simulink model "Modulador_Analogico_CuatroUsuarios"  (R2018b)
settings: Solver=FixedStepAuto  StartTime=0.0  StopTime=M*CantBit  FixedStep=Tsampling  RelTol=1e-3
values from neighbouring files (symbols this model uses):
  CantMPerSimbOFDM = round(TsOFDM/Tsampling)    [Script_configParametros.m]
  EsOFDM = 2    [Script_configParametros.m]
  F1 = FsepOFDM*2    [Script_configParametros.m]
  F2 = FsepOFDM*3    [Script_configParametros.m]
  F3 = FsepOFDM*4    [Script_configParametros.m]
  F4 = FsepOFDM*5    [Script_configParametros.m]
  Tb1 = 1/Rb1    (= 0.001)    [Script_configParametros.m]
  Tb2 = 1/Rb2    (= 0.001)    [Script_configParametros.m]
  Tb3 = 1/Rb3    (= 0.0005)    [Script_configParametros.m]
  Tb4 = 1/Rb4    (= 0.000333333333333)    [Script_configParametros.m]
  Ts1 = Tb1    (= 0.001)    [Script_configParametros.m]
  Ts2 = Tb2    (= 0.001)    [Script_configParametros.m]
  Ts3 = 2*Tb3    (= 0.001)    [Script_configParametros.m]
  Ts4 = 3*Tb4    (= 0.001)    [Script_configParametros.m]
  Tsampling = M/N    [Script_configParametros.m]
libraries: commdigbbndpm3 x4, commrandsrc3 x4
settings Model: Creator=lukit  LastModifiedBy=lukit

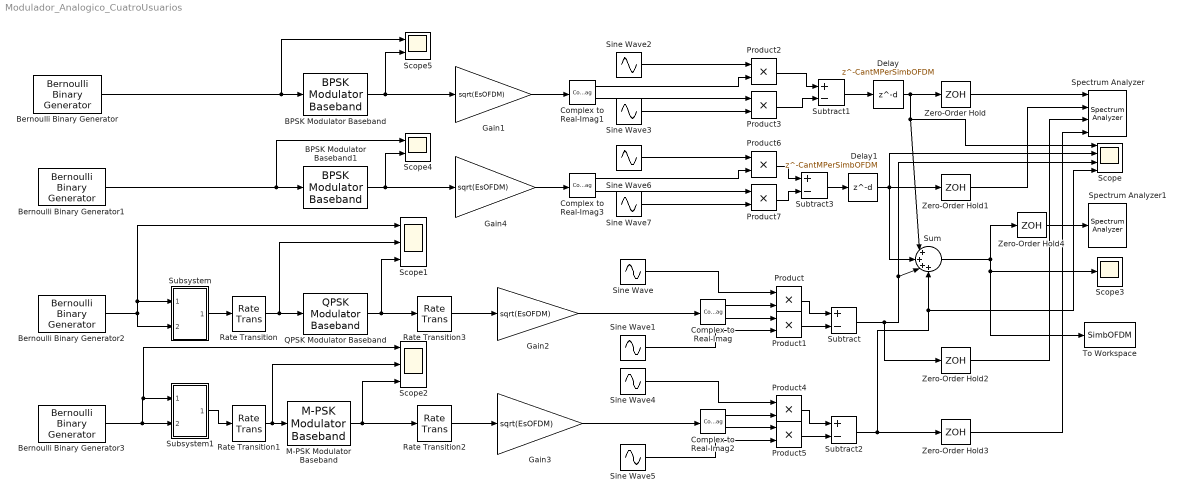
== system Modulador_Analogico_CuatroUsuarios ==
  BPSK Modulator Baseband : commdigbbndpm3/BPSK Modulator Baseband  Ph=0  outDtype=double  outWordLen=16  outUDDataType=sfix(16)  outFracLenMode=Best precision  outFracLen=15  outDataTypeStr=double  outLastDataTypeStr=double
  BPSK Modulator Baseband1 : commdigbbndpm3/BPSK Modulator Baseband  Ph=0  outDtype=double  outWordLen=16  outUDDataType=sfix(16)  outFracLenMode=Best precision  outFracLen=15  outDataTypeStr=double  outLastDataTypeStr=double
  Bernoulli Binary Generator : commrandsrc3/Bernoulli Binary Generator  ProbabilityOfZero=0.5  SeedSource=Auto  Seed=0  SampleTime=Tb1  SamplesPerFrame=1  OutputDataType=double  SimulateUsing=Interpreted execution
  Bernoulli Binary Generator1 : commrandsrc3/Bernoulli Binary Generator  ProbabilityOfZero=0.5  SeedSource=Auto  Seed=0  SampleTime=Tb2  SamplesPerFrame=1  OutputDataType=double  SimulateUsing=Interpreted execution
  Bernoulli Binary Generator2 : commrandsrc3/Bernoulli Binary Generator  ProbabilityOfZero=0.5  SeedSource=Auto  Seed=0  SampleTime=Tb3  SamplesPerFrame=1  OutputDataType=double  SimulateUsing=Interpreted execution
  Bernoulli Binary Generator3 : commrandsrc3/Bernoulli Binary Generator  ProbabilityOfZero=0.5  SeedSource=Auto  Seed=0  SampleTime=Tb4  SamplesPerFrame=1  OutputDataType=double  SimulateUsing=Interpreted execution
  Complex to Real-Imag{,1..3} (4 alike) : ComplexToRealImag
  Delay : Delay  DelayLength=CantMPerSimbOFDM  InitialCondition=0  SampleTime=Tsampling
  Delay1 : Delay  DelayLength=CantMPerSimbOFDM  InitialCondition=0  SampleTime=Tsampling
  Gain{1..4} (4 alike) : Gain  Gain=sqrt(EsOFDM)
  M-PSK Modulator Baseband : commdigbbndpm3/M-PSK Modulator Baseband  M=8  InType=Integer  Enc=Gray  Mapping=[0:7]  Ph=0  outDtype=double  outWordLen=16  outUDDataType=sfix(16)  outFracLenMode=Best precision  outFracLen=15  outDataTypeStr=double  outLastDataTypeStr=double
      settings: SourceProductName=Communications System Toolbox
  Product{,1..7} (8 alike) : Product
  QPSK Modulator Baseband : commdigbbndpm3/QPSK Modulator Baseband  InType=Integer  Enc=Gray  Ph=0  outDtype=double  outWordLen=16  outUDDataType=sfix(16)  outFracLenMode=Best precision  outFracLen=15  outDataTypeStr=double  outLastDataTypeStr=double
  Rate Transition : RateTransition  OutPortSampleTime=Ts3
  Rate Transition1 : RateTransition  OutPortSampleTime=Ts4
  Rate Transition2 : RateTransition  OutPortSampleTime=Tsampling
  Rate Transition3 : RateTransition  OutPortSampleTime=Tsampling
  Scope : Scope  NumInputPorts=4
  Scope1 : Scope  NumInputPorts=3
  Scope2 : Scope  NumInputPorts=3
  Scope3 : Scope
  Scope4 : Scope  NumInputPorts=2
  Scope5 : Scope  NumInputPorts=2
  Sine Wave : Sin  Amplitude=sqrt(2/Ts3)  Frequency=2*pi*F3  Phase=pi/2  SampleTime=Tsampling
  Sine Wave1 : Sin  Amplitude=sqrt(2/Ts3)  Frequency=2*pi*F3  SampleTime=Tsampling
  Sine Wave2 : Sin  Amplitude=sqrt(2/Ts1)  Frequency=2*pi*F1  Phase=pi/2  SampleTime=Tsampling
  Sine Wave3 : Sin  Amplitude=sqrt(2/Ts1)  Frequency=2*pi*F1  SampleTime=Tsampling
  Sine Wave4 : Sin  Amplitude=sqrt(2/Ts4)  Frequency=2*pi*F4  Phase=pi/2  SampleTime=Tsampling
  Sine Wave5 : Sin  Amplitude=sqrt(2/Ts4)  Frequency=2*pi*F4  SampleTime=Tsampling
  Sine Wave6 : Sin  Amplitude=sqrt(2/Ts2)  Frequency=2*pi*F2  Phase=pi/2  SampleTime=Tsampling
  Sine Wave7 : Sin  Amplitude=sqrt(2/Ts2)  Frequency=2*pi*F2  SampleTime=Tsampling
  Spectrum Analyzer : SpectrumAnalyzer  NumInputPorts=4
  Spectrum Analyzer1 : SpectrumAnalyzer
  Subsystem : Subsystem
  Subsystem1 : Subsystem
  Subtract{,1..3} (4 alike) : Sum  Inputs=+-
  Sum : Sum  Inputs=|++++
  To Workspace : ToWorkspace  VariableName=SimbOFDM  SampleTime=Tsampling
      settings: Save2DSignal=2-D array (concatenate along first dimension)
  Zero-Order Hold{,1..4} (5 alike) : ZeroOrderHold  SampleTime=-1
  wires:
  Product/1 -> Subtract/1
  Product1/1 -> Subtract/2
  Sine Wave/1 -> Product/1
  Sine Wave1/1 -> Product1/2
  Complex to Real-Imag/2 -> Product1/1
  Complex to Real-Imag/1 -> Product/2
  Gain2/1 -> Complex to Real-Imag/1
  Bernoulli Binary Generator/1 -> Scope5/1, BPSK Modulator Baseband/1
  Sine Wave2/1 -> Product2/1
  Complex to Real-Imag1/1 -> Product2/2
  Sine Wave3/1 -> Product3/2
  Complex to Real-Imag1/2 -> Product3/1
  Gain1/1 -> Complex to Real-Imag1/1
  Product2/1 -> Subtract1/1
  Product3/1 -> Subtract1/2
  BPSK Modulator Baseband/1 -> Scope5/2, Gain1/1
  Subtract/1 -> Zero-Order Hold2/1, Scope/3, Sum/3
  QPSK Modulator Baseband/1 -> Rate Transition3/1, Scope1/3
  M-PSK Modulator Baseband/1 -> Scope2/3, Rate Transition2/1
  Product4/1 -> Subtract2/1
  Sine Wave4/1 -> Product4/1
  Product5/1 -> Subtract2/2
  Sine Wave5/1 -> Product5/2
  Subtract2/1 -> Zero-Order Hold3/1, Scope/4, Sum/4
  Complex to Real-Imag2/2 -> Product5/1
  Complex to Real-Imag2/1 -> Product4/2
  Gain3/1 -> Complex to Real-Imag2/1
  Bernoulli Binary Generator1/1 -> Scope4/1, BPSK Modulator Baseband1/1
  BPSK Modulator Baseband1/1 -> Scope4/2, Gain4/1
  Sine Wave6/1 -> Product6/1
  Complex to Real-Imag3/1 -> Product6/2
  Sine Wave7/1 -> Product7/2
  Product6/1 -> Subtract3/1
  Product7/1 -> Subtract3/2
  Complex to Real-Imag3/2 -> Product7/1
  Gain4/1 -> Complex to Real-Imag3/1
  Subtract3/1 -> Delay1/1
  Sum/1 -> To Workspace/1, Scope3/1, Zero-Order Hold4/1
  Zero-Order Hold/1 -> Spectrum Analyzer/1
  Zero-Order Hold1/1 -> Spectrum Analyzer/2
  Zero-Order Hold2/1 -> Spectrum Analyzer/3
  Zero-Order Hold3/1 -> Spectrum Analyzer/4
  Zero-Order Hold4/1 -> Spectrum Analyzer1/1
  Bernoulli Binary Generator2/1 -> Subsystem/2(In2), Scope1/1, Subsystem/1(In1)
  Rate Transition/1 -> Scope1/2, QPSK Modulator Baseband/1
  Subsystem/1(Out1) -> Rate Transition/1
  Bernoulli Binary Generator3/1 -> Scope2/1, Subsystem1/1(In1), Subsystem1/2(In2)
  Rate Transition1/1 -> Scope2/2, M-PSK Modulator Baseband/1
  Subsystem1/1(Out1) -> Rate Transition1/1
  Rate Transition2/1 -> Gain3/1
  Rate Transition3/1 -> Gain2/1
  Subtract1/1 -> Delay/1
  Delay1/1 -> Zero-Order Hold1/1, Sum/2, Scope/2
  Delay/1 -> Sum/1, Scope/1, Zero-Order Hold/1

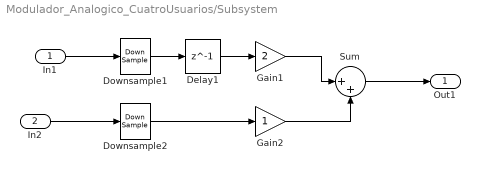
== system Modulador_Analogico_CuatroUsuarios/Subsystem ==
  In1 : Inport
  In2 : Inport  Port=2
  Delay1 : Delay  DelayLength=1  InitialCondition=0
  Downsample1 : DownSample  RateOptions=Allow multirate processing
  Downsample2 : DownSample  phase=1  RateOptions=Allow multirate processing
  Gain1 : Gain  Gain=2
  Gain2 : Gain
  Sum : Sum  Inputs=|++
  Out1 : Outport
  wires:
  Gain1/1 -> Sum/1
  Downsample2/1 -> Gain2/1
  Sum/1 -> Out1/1
  Downsample1/1 -> Delay1/1
  Delay1/1 -> Gain1/1
  Gain2/1 -> Sum/2
  In2/1 -> Downsample2/1
  In1/1 -> Downsample1/1

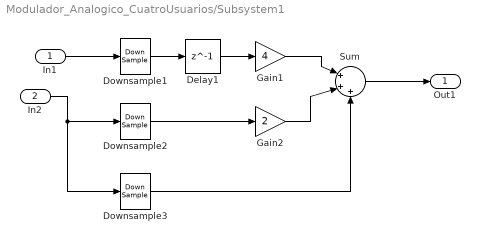
== system Modulador_Analogico_CuatroUsuarios/Subsystem1 ==
  In1 : Inport
  In2 : Inport  Port=2
  Delay1 : Delay  DelayLength=1  InitialCondition=0
  Downsample1 : DownSample  N=3  RateOptions=Allow multirate processing
  Downsample2 : DownSample  N=3  phase=1  RateOptions=Allow multirate processing
  Downsample3 : DownSample  N=3  phase=2  RateOptions=Allow multirate processing
  Gain1 : Gain  Gain=4
  Gain2 : Gain  Gain=2
  Sum : Sum  Inputs=|+++
  Out1 : Outport
  wires:
  Gain1/1 -> Sum/1
  Downsample2/1 -> Gain2/1
  Sum/1 -> Out1/1
  Downsample1/1 -> Delay1/1
  Delay1/1 -> Gain1/1
  Gain2/1 -> Sum/2
  In2/1 -> Downsample3/1, Downsample2/1
  Downsample3/1 -> Sum/3
  In1/1 -> Downsample1/1
